simulink model "ifft_tut"  (Simulink 4.00)
settings: Solver=FixedStepDiscrete  StartTime=0.0  StopTime=inf  RelTol=1e-3
PostLoadFcn:
  | set_param(gcs,'SimulationCommand','Update')
undefined symbols (not defined in the file or in its folder): get
libraries: dspxfrm3 x2, dspmtrx3 x1, dspsrcs3 x1, dspsnks3 x1
settings Model: RequirementInfo=9  Creator=ckamachi  LastModifiedBy=ckamachi  LimitDataPoints=off  ExtModeTrigMode=oneshot  ExtModeArmWhenConnect=off  BlockReductionOpt=off

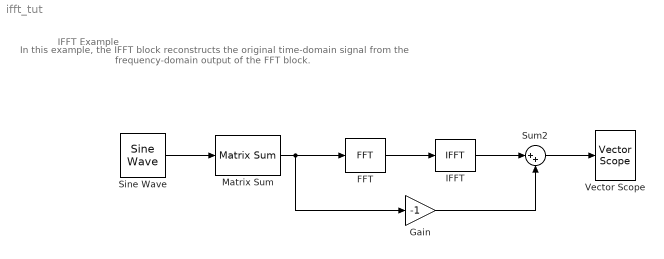
== system ifft_tut ==
  note: IFFT Example
  note: In this example, the IFFT block reconstructs the original time-domain signal from the
      | frequency-domain output of the FFT block.
  FFT : dspxfrm3/FFT  CompMethod=Table lookup  TableOpt=Speed  BitRevOrder=on
  Gain : Gain  Gain=-1  Multiplication=Element-wise(K.*u)  SaturateOnIntegerOverflow=on
  IFFT : dspxfrm3/IFFT  CompMethod=Table lookup  TableOpt=Speed  BitRevOrder=on  cs_in=on  SkipNorm=off  mode=Real
  Matrix Sum : dspmtrx3/Matrix Sum  Dim=Rows
  Sine Wave : dspsrcs3/Sine Wave  Amplitude=1  Frequency=[15 40]  Phase=0  SampleMode=Discrete  OutComplex=Real  CompMethod=Trigonometric Fcn  TableSize=Speed  SampleTime=0.001  SamplesPerFrame=128  ResetState=Restart at time zero
  Sum2 : Sum  Inputs=|++  SaturateOnIntegerOverflow=on
  Vector Scope : dspsnks3/Vector Scope  ScopeProperties=on  Domain=Time  HorizSpan=1  DisplayProperties=off  AxisGrid=on  Memory=off  FrameNumber=on  AxisLegend=off  AxisZoom=off  OpenScopeAtSimStart=on  OpenScopeImmediately=off  FigPos=get(0,'defaultfigureposition')  AxisProperties=off  XUnits=Hertz  XRange=[0...Fs/2]  InheritXIncr=on  XIncr=1  XLabel=Samples  YUnits=dB  YLabel=Amplitude  LineProperties=off
      settings: YMin=-10  YMax=10
  wires:
  Sine Wave/1 -> Matrix Sum/1
  Matrix Sum/1 -> FFT/1, Gain/1
  FFT/1 -> IFFT/1
  Gain/1 -> Sum2/2
  IFFT/1 -> Sum2/1
  Sum2/1 -> Vector Scope/1
